simulink model "TIntkVUs_VD"  (R2016b)
settings: configuration reference "CodeGenConfigSet" (kept outside this file)
values from neighbouring files (symbols this model uses):
  Air_facPT1TIntkVUs_C = Calibration.Parameter    [init_TIntkVUs_VD.m]
  Air_RmpSlpTIntkVUsNeg_C = Calibration.Parameter    [init_TIntkVUs_VD.m]
  Air_RmpSlpTIntkVUsPos_C = Calibration.Parameter    [init_TIntkVUs_VD.m]
  Air_tTransStgTIntkVUsDfl_C = Calibration.Parameter    [init_TIntkVUs_VD.m]
  SigTst_swtTIntkVUs_C = Calibration.Parameter    [init_TIntkVUs_VD.m]
  SigTst_tIntkVUs_C = Calibration.Parameter    [init_TIntkVUs_VD.m]
undefined symbols (not defined in the file or in its folder): CEngDst_switch_conv, Switch_conv, TIntkVUs_VD_DT
libraries: CXLib x4
settings Model: Creator=GaberXu  LastModifiedBy=zhoutinglin
settings ConfigSetRef: SourceLocation=Base Workspace

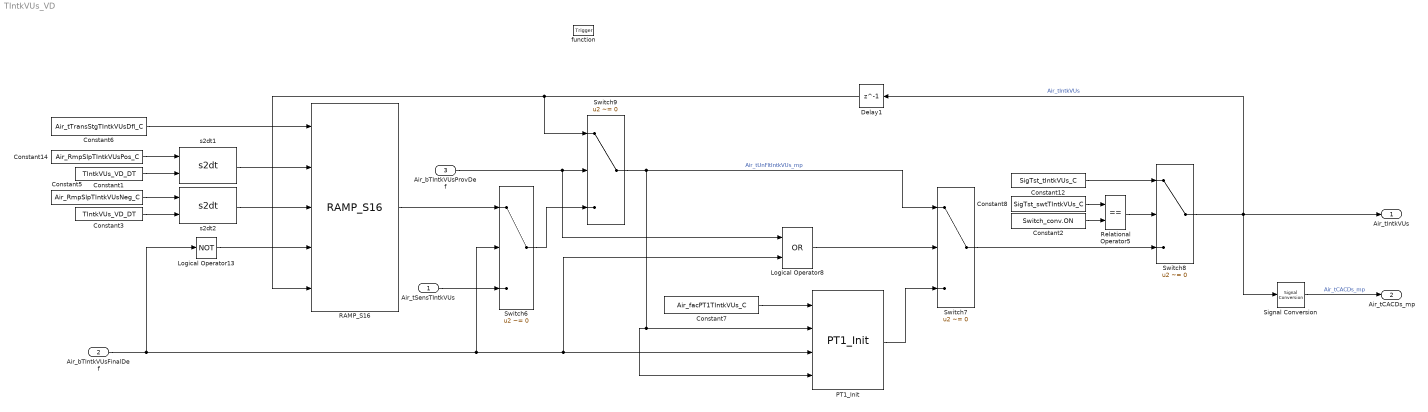
== system TIntkVUs_VD ==
  Air_tSensTIntkVUs : Inport  Tag=deg  Description=Sensed value of air temperature upstream of the intake valve  OutMin=-200  OutMax=200  OutDataTypeStr=Temp_deg
  Air_bTIntkVUsFinalDef : Inport  Description=Final defect of the raw air temperature upstream of the intake valve  Port=2  OutMin=0  OutMax=1  OutDataTypeStr=boolean
  Air_bTIntkVUsProvDef : Inport  Description=Provisional defect of the raw air temperature upstream of the intake valve  Port=3  OutMin=0  OutMax=1  OutDataTypeStr=boolean
  function : TriggerPort  TriggerType=function-call  VariantControl=Variant
  Constant1 : Constant  Value=TIntkVUs_VD_DT  SampleTime=-1
  Constant12 : Constant  RequirementInfo={'other' 'CEngDsT_requirements.doc' '@Simulink_requirement_item_6' 'true' '手动冷却水温值' '' } %GIDa_73e2ab8d_4bbe_45bd_8127_2162d48852d3  Value=SigTst_tIntkVUs_C  SampleTime=-1
  Constant14 : Constant  RequirementInfo={'other' 'CEngDsT_requirements.doc' '@Simulink_requirement_item_8' 'true' '冷却水温故障时斜坡至默认值' '' } %GIDa_bd091f41_5138_410e_abb6_2bd2d1e5c8b0  Value=Air_RmpSlpTIntkVUsPos_C  SampleTime=-1
  Constant2 : Constant  RequirementInfo={'other' 'APP_requirements.doc' '@Simulink_requirement_item_25' 'true' '手动开关' '' } %GIDa_0ae123b2_a266_4b86_a827_c8b3943914da  Value=Switch_conv.ON  OutDataTypeStr=Inherit: Inherit via back propagation
  Constant3 : Constant  Value=TIntkVUs_VD_DT  SampleTime=-1
  Constant5 : Constant  RequirementInfo={'other' 'CEngDsT_requirements.doc' '@Simulink_requirement_item_8' 'true' '冷却水温故障时斜坡至默认值' '' } %GIDa_9b768724_a4eb_43d2_8305_93f4e5b79678  Value=Air_RmpSlpTIntkVUsNeg_C  SampleTime=-1
  Constant6 : Constant  RequirementInfo={'other' 'CEngDsT_requirements.doc' '@Simulink_requirement_item_8' 'true' '冷却水温故障时斜坡至默认值' '' } %GIDa_d761315b_10ec_40e2_ad8e_ad829b48c1b7  Value=Air_tTransStgTIntkVUsDfl_C  SampleTime=-1
  Constant7 : Constant  Value=Air_facPT1TIntkVUs_C  SampleTime=-1
  Constant8 : Constant  RequirementInfo={'other' 'CEngDsT_requirements.doc' '@Simulink_requirement_item_6' 'true' '手动冷却水温值' '' } %GIDa_9b1f3048_f79a_4d31_ad90_183e1d10eb7d  Value=SigTst_swtTIntkVUs_C  SampleTime=-1
  Delay1 : Delay  DialogController=Simulink.DDGSource  DelayLength=1  InitialCondition=0
  Logical Operator13 : Logic  Operator=NOT  AllPortsSameDT=off  OutDataTypeStr=boolean
  Logical Operator8 : Logic  Operator=OR  OutDataTypeStr=boolean
  PT1_Init : CXLib/PT1_Init
  RAMP_S16 : CXLib/RAMP_S16  RequirementInfo={'other' 'CEngDsT_requirements.doc' '@Simulink_requirement_item_8' 'true' '冷却水温故障时斜坡至默认值' '' } %GIDa_f2fde6ef_f087_4cf6_87f7_1e63c9d60487
  Relational Operator5 : RelationalOperator  Operator===  OutDataTypeStr=boolean  RndMeth=Simplest  InputSameDT=on
  Signal Conversion : SignalConversion  OverrideOpt=off
  Switch6 : Switch  Criteria=u2 ~= 0  InputSameDT=on
  Switch7 : Switch  RequirementInfo={'other' 'CEngDsT_requirements.doc' '@Simulink_requirement_item_5' 'true' '冷却水温滤波去抖动' '' } %GIDa_a6bfae42_32d3_49b5_ad25_923501f4b963  Criteria=u2 ~= 0  InputSameDT=on
  Switch8 : Switch  RequirementInfo={'other' 'CEngDsT_requirements.doc' '@Simulink_requirement_item_6' 'true' '手动冷却水温值' '' } %GIDa_01c4b358_7c94_4f03_b18c_60ec62b27b4c  Criteria=u2 ~= 0  Threshold=CEngDst_switch_conv.OFF  InputSameDT=on
  Switch9 : Switch  Criteria=u2 ~= 0  InputSameDT=on
  s2dt1 : CXLib/s2dt
  s2dt2 : CXLib/s2dt
  Air_tIntkVUs : Outport  Tag=deg  Description=Intake air temperature upstream of the inlet valve  OutMin=-200  OutMax=200  OutDataTypeStr=Temp_deg
  Air_tCACDs_mp : Outport  Tag=deg  Description=Charge-air temperature downstream from charge-air cooler  Port=2  OutMin=-200  OutMax=200  OutDataTypeStr=Temp_deg
  wires:
  Switch9/1 -> PT1_Init/4, PT1_Init/2, Switch7/1  "Air_tUnFltIntkVUs_mp"
  Switch6/1 -> Switch9/3
  Logical Operator8/1 -> Switch7/2
  Switch7/1 -> Switch8/3
  Switch8/1 -> Air_tIntkVUs/1, Delay1/1, Signal Conversion/1  "Air_tIntkVUs"
  Constant6/1 -> RAMP_S16/1
  Logical Operator13/1 -> RAMP_S16/4
  Constant12/1 -> Switch8/1
  Constant7/1 -> PT1_Init/1
  RAMP_S16/1 -> Switch6/1
  PT1_Init/1 -> Switch7/3
  Air_bTIntkVUsFinalDef/1 -> Logical Operator13/1, PT1_Init/3, Logical Operator8/2, Switch6/2
  Air_bTIntkVUsProvDef/1 -> Logical Operator8/1, Switch9/2
  Relational Operator5/1 -> Switch8/2
  Constant8/1 -> Relational Operator5/1
  Constant2/1 -> Relational Operator5/2
  Delay1/1 -> Switch9/1, RAMP_S16/5
  Constant14/1 -> s2dt1/1
  Constant1/1 -> s2dt1/2
  s2dt1/1 -> RAMP_S16/2
  Constant5/1 -> s2dt2/1
  Constant3/1 -> s2dt2/2
  s2dt2/1 -> RAMP_S16/3
  Air_tSensTIntkVUs/1 -> Switch6/3
  Signal Conversion/1 -> Air_tCACDs_mp/1  "Air_tCACDs_mp"
